simulink library "Lib_Solve_SSNRSolverJC_TMATS"  (R2012b)
settings: Solver=ode45  StartTime=0.0  StopTime=10.0  RelTol=1e-3
libraries: Lib_NM_JacobianCalc_TMATS x1, Lib_NM_NewtonRaphsonSolver_TMATS x1
Description:
  | Thomas Modules
settings Model: Creator=jwchapm2  LastModifiedBy=jwchapm2

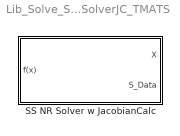
== system Lib_Solve_SSNRSolverJC_TMATS ==
  SS NR Solver w JacobianCalc : Subsystem  mask(T-MATS: SS NR Solver w Jacobian Calc Library Block){SJac_Per_M=[0.01; 0.05; 0.05], SNR_IC_M=[1 2 3], SNR_DX_M=5, SJacobianAttempts_M=20, Cond_Limits_M=0.1}
      mask prompts: SJac_Per_M "SJac_Per_M - Jacobian Perturbation size (frac)(nx1)"; SNR_IC_M "SNR_IC_M - Newton Raphson Initial Conditions (nx1)"; SNR_DX_M "SNR_DX_M - Newton Raphson delta x limiter (%) (1x1)"; SJacobianAttempts_M "SJacobianAttempts_M - Newton Raphson attempts before the Jacobian recalculation (1x1)"; Cond_Limits_M "Cond_Limits_M - Iteration Conditions Limits (nx1 or 1x1)"
      mask help:
      | The Steady State Newton Raphson Solver with Jacobian Calculator block will
      | supply the inputs to iteratively drive the outputs of a system to zero.
      |
      | This will be performed in three steps.
      | 1) Jabobian calculator sends Perturbations to the plant then calculates the plant
      | Jacboian based on the system response
      | 2) The Newton Raphson will use the inverse of the Jacobian to iteratively step the
      | system toward solution.
      | 3) Once the solution has satisfied the conditions the Newton Raphson is shut off.
      |
      | Simulation run time length should be selected as to give the Newton Raphson solver adequate time to develop a solution.
      mask Help: web(which('Solver_TMATS_SSNRwJC.html'),'-helpbrowser')

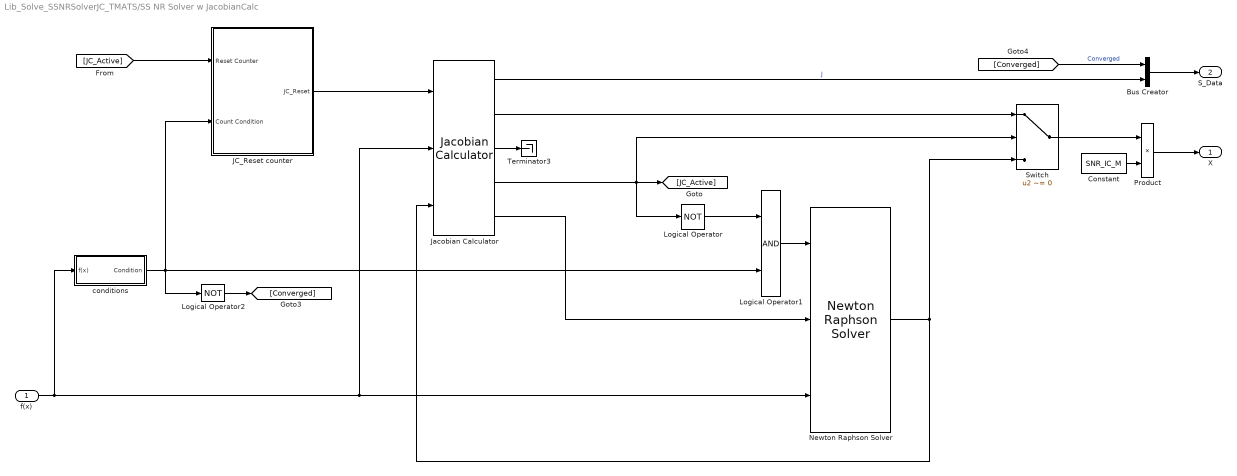
== system Lib_Solve_SSNRSolverJC_TMATS/SS NR Solver w JacobianCalc ==
  f(x) : Inport
  Bus Creator : BusCreator  Inputs=2
  Constant : Constant  Value=SNR_IC_M
  JC_Reset counter : Subsystem
  Jacobian Calculator : Lib_NM_JacobianCalc_TMATS/Jacobian Calculator  N_Per_M=SJac_Per_M
  Logical Operator : Logic  Operator=NOT  AllPortsSameDT=off  OutDataTypeStr=boolean
  Logical Operator1 : Logic  AllPortsSameDT=off  OutDataTypeStr=boolean
  Logical Operator2 : Logic  Operator=NOT  AllPortsSameDT=off  OutDataTypeStr=boolean
  Newton Raphson Solver : Lib_NM_NewtonRaphsonSolver_TMATS/Newton Raphson Solver  NR_IC_M=ones(length(SNR_IC_M),1)  NR_dx_Lim_M=SNR_DX_M
  Product : Product  RndMeth=Zero
  Switch : Switch  Criteria=u2 ~= 0  Threshold=1
  Terminator3 : Terminator
  conditions : Subsystem
  X : Outport
  S_Data : Outport  Port=2
  wires:
  Logical Operator1/1 -> Newton Raphson Solver/1
  Logical Operator/1 -> Logical Operator1/1
  Jacobian Calculator/4 -> Switch/2, [JC_Active], Logical Operator/1
  Jacobian Calculator/1 -> Bus Creator/2  "J"
  Jacobian Calculator/2 -> Switch/1
  Jacobian Calculator/5 -> Newton Raphson Solver/2
  Newton Raphson Solver/1 -> Jacobian Calculator/3, Switch/3
  Jacobian Calculator/3 -> Terminator3/1
  f(x)/1 -> conditions/1(f(x)), Newton Raphson Solver/3, Jacobian Calculator/2
  conditions/1(Condition) -> Logical Operator2/1, JC_Reset counter/2(Count Condition), Logical Operator1/2
  JC_Reset counter/1(JC_Reset) -> Jacobian Calculator/1
  [JC_Active] -> JC_Reset counter/1(Reset Counter)
  Switch/1 -> Product/1
  Product/1 -> X/1
  Constant/1 -> Product/2
  Logical Operator2/1 -> [Converged]
  [Converged] -> Bus Creator/1  "Converged"
  Bus Creator/1 -> S_Data/1

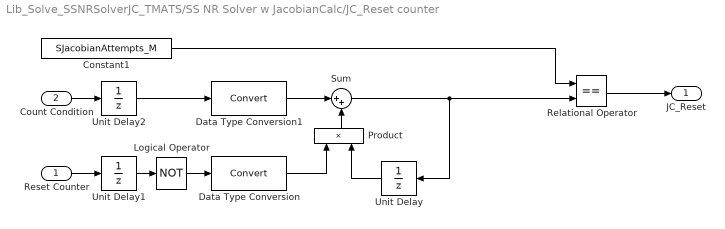
== system Lib_Solve_SSNRSolverJC_TMATS/SS NR Solver w JacobianCalc/JC_Reset counter ==
  Reset Counter : Inport
  Count Condition : Inport  Port=2
  Constant1 : Constant  Value=SJacobianAttempts_M
  Data Type Conversion : DataTypeConversion
  Data Type Conversion1 : DataTypeConversion
  Logical Operator : Logic  Operator=NOT  AllPortsSameDT=off  OutDataTypeStr=boolean
  Product : Product  RndMeth=Zero
  Relational Operator : RelationalOperator  Operator===  OutDataTypeStr=boolean
  Sum : Sum  Inputs=|++
  Unit Delay : UnitDelay  SampleTime=-1
  Unit Delay1 : UnitDelay  SampleTime=-1
  Unit Delay2 : UnitDelay  SampleTime=-1
  JC_Reset : Outport
  wires:
  Constant1/1 -> Relational Operator/1
  Relational Operator/1 -> JC_Reset/1
  Product/1 -> Sum/2
  Reset Counter/1 -> Unit Delay1/1
  Unit Delay/1 -> Product/2
  Data Type Conversion/1 -> Product/1
  Data Type Conversion1/1 -> Sum/1
  Unit Delay1/1 -> Logical Operator/1
  Logical Operator/1 -> Data Type Conversion/1
  Count Condition/1 -> Unit Delay2/1
  Unit Delay2/1 -> Data Type Conversion1/1
  Sum/1 -> Unit Delay/1, Relational Operator/2

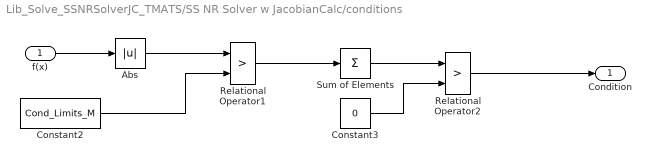
== system Lib_Solve_SSNRSolverJC_TMATS/SS NR Solver w JacobianCalc/conditions ==
  f(x) : Inport
  Abs : Abs
  Constant2 : Constant  Value=Cond_Limits_M
  Constant3 : Constant  Value=0
  Relational Operator1 : RelationalOperator  Operator=>  OutDataTypeStr=boolean
  Relational Operator2 : RelationalOperator  Operator=>  OutDataTypeStr=boolean
  Sum of Elements : Sum  Inputs=+
  Condition : Outport
  wires:
  Constant2/1 -> Relational Operator1/2
  Relational Operator1/1 -> Sum of Elements/1
  Constant3/1 -> Relational Operator2/2
  Abs/1 -> Relational Operator1/1
  Sum of Elements/1 -> Relational Operator2/1
  f(x)/1 -> Abs/1
  Relational Operator2/1 -> Condition/1
